simulink model "Flyback75W"  (R2019a)
settings: Solver=VariableStepAuto  StartTime=0.0  StopTime=.05  RelTol=1e-3
libraries: powerlib x21, powerlib_meascontrol x1, simulink x1
settings Model: Creator=victor  LastModifiedBy=victor

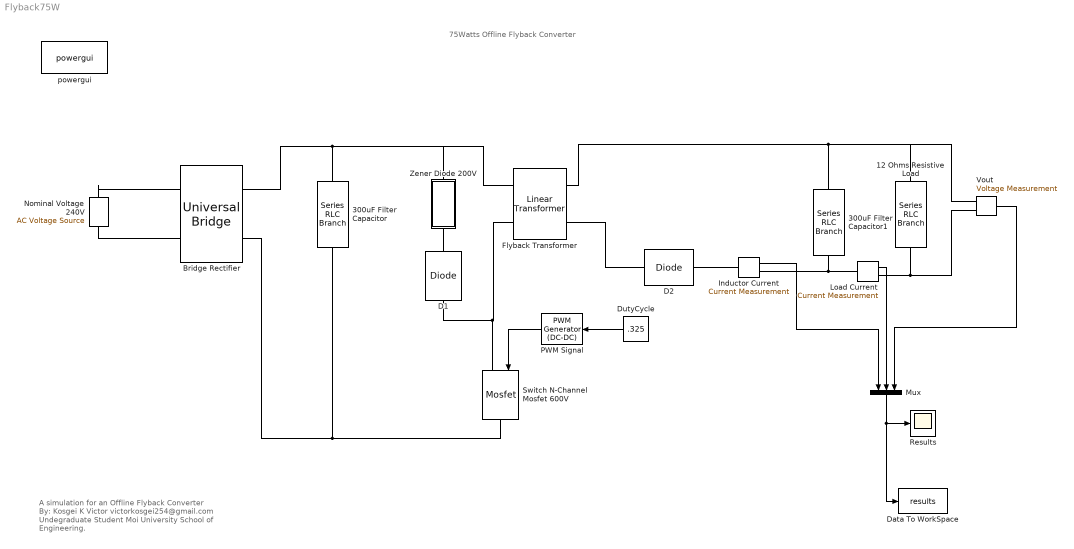
== system Flyback75W ==
  note: 75Watts Offline Flyback Converter
  note: A simulation for an Offline Flyback Converter
      | By: Kosgei K Victor
      | 	victorkosgei254@gmail.com
      | 	Undegraduate Student
      | 	Moi University
      | 	School of Engineering.
  12 Ohms Resistive Load : powerlib/Elements/Series RLC Branch  LConnTagsString=__new0  RConnTagsString=__new0  BranchType=R  Resistance=12  Inductance=1e-3  SetiL0=off  InitialCurrent=0  Capacitance=1e-6  Setx0=off  InitialVoltage=0  Measurements=None
      settings: SourceProductName=Simscape Electrical
  300uF Filter Capacitor : powerlib/Elements/Series RLC Branch  LConnTagsString=__new0  RConnTagsString=__new0  BranchType=C  Resistance=1  Inductance=1e-3  SetiL0=off  InitialCurrent=0  Capacitance=300e-6  Setx0=off  InitialVoltage=0  Measurements=None
      settings: SourceProductName=Simscape Electrical
  300uF Filter Capacitor1 : powerlib/Elements/Series RLC Branch  LConnTagsString=__new0  RConnTagsString=__new0  BranchType=C  Resistance=1  Inductance=1e-3  SetiL0=off  InitialCurrent=0  Capacitance=300e-6  Setx0=off  InitialVoltage=0  Measurements=None
      settings: SourceProductName=Simscape Electrical
  Bridge Rectifier : powerlib/Power Electronics/Universal Bridge  Arms=2  SnubberResistance=1e5  SnubberCapacitance=inf  Device=Diodes  Ron=1e-3  Lon=0  ForwardVoltages="[  0  0  ]"  ForwardVoltage=0  GTOparameters=[ 10e-6 , 20e-6 ]  IGBTparameters=[ 1e-6 , 2e-6 ]  Measurements=None  Measurements_2=None  converterType=Rectifier
      settings: SourceProductName=Simscape Electrical
  D1 : powerlib/Power Electronics/Diode  Ron=0.001  Lon=0  Vf=0.8  IC=0  UseSnubber=0  Rs=500  Cs=250e-9  Measurements=off
      settings: SourceProductName=Simscape Electrical
  D2 : powerlib/Power Electronics/Diode  Ron=0.001  Lon=0  Vf=0.8  IC=0  UseSnubber=0  Rs=500  Cs=250e-9  Measurements=off
      settings: SourceProductName=Simscape Electrical
  Data To WorkSpace : ToWorkspace  VariableName=results  SaveFormat=Timeseries  SampleTime=-1
  DutyCycle : Constant  Value=.325
  Flyback Transformer : powerlib/Elements/Linear Transformer  UNITS=SI  NominalPower=[ 84 250e3 ]  winding1=[540 0 833.9e-6]  winding2=[21.2 0 8.75e-6]  ThreeWindings=off  winding3=[3.15e+05 2.3625e+06 60.161]  RmLm=[3.2156e+12 68.336e-9]  Measurements=None  DataType=on
      settings: SourceProductName=Simscape Electrical
  Inductor Current : powerlib/Measurements/Current Measurement  PhasorSimulation=off  OutputType=Complex  PSBequivalent=0
      settings: SourceProductName=Simscape Electrical
  "Load Current " : powerlib/Measurements/Current Measurement  PhasorSimulation=off  OutputType=Complex  PSBequivalent=0
      settings: SourceProductName=Simscape Electrical
  Mux : Mux  Inputs=3
  Nominal Voltage 240V : powerlib/Electrical Sources/AC Voltage Source  Amplitude=100  Phase=0  Frequency=60  SampleTime=0  Measurements=None  BusType=swing  Pref=10e3  Qref=0  Qmin=-inf  Qmax=+inf
      settings: SourceProductName=Simscape Electrical
  PWM Signal : powerlib_meascontrol/Pulse & Signal Generators/PWM Generator (DC-DC)  Fsw=5000  Ts=0
      settings: SourceProductName=Simscape Electrical
  "Results " : Scope
  Switch N-Channel Mosfet 600V : powerlib/Power Electronics/Mosfet  Ron=0.1  Lon=0  Rd=0.01  Vfd=0  IC=0  Rs=1e5  Cs=inf  Measurements=off
      settings: SourceProductName=Simscape Electrical
  Vout : powerlib/Measurements/Voltage Measurement  PhasorSimulation=off  OutputType=Complex  PSBequivalent=0
      settings: SourceProductName=Simscape Electrical
  Zener Diode 200V : Subsystem  mask(Zener Diode){Vz=10, Rzt=10, Rzk=400, Izm=400e-3, Vf=0.7, Ron=1e-3}
      mask prompts: Vz "Zener Voltage Vz (V)"; Rzt "Dynamic Impedance Zzt (ohms)"; Rzk "Knee Impedance Zzk (ohms)"; Izm "Maximum Continuous Current Izm (A)"; Vf "Forward Voltage Drop Vf (V)"; Ron "On Resistance Ron (ohms)"
      mask help:
      | Implements a zener diode block.
      | Use values from standard datasheets to populate block dialog
  powergui : powerlib/powergui  Priority=1  SimulationMode=Discrete  SampleTime=1e-6  frequency=60  Iterations=50  frequencyindice=60  Pbase=100e6  ErrMax=1e-4  UnitsV=kV  UnitsW=MW  buscounter=0  FunctionMessages=off  echomessages=off  EnableUseOfTLC=off  CurrentSourceSwitches=off  DisableSnubberDevices=off  DisableRonSwitches=off  DisableVfSwitches=off  DisplayEquations=off  AutomaticDiscreteSolvers=off  SolverType=Tustin/Backward Euler (TBE)  Interpol=off  ExternalGateDelay=off  methode=off  Ts=100  x0status=blocks  SPID=on  SwTol=0  HookPort=off  NonlinearTolerance=0  nMaxIteration=15  ContinueOnMaxIteration=off  RestoreLinks=warning  ResistiveCurrentMeasurement=off  Frange=[0:2:500]  Ylog=off  Xlog=on  ShowGrid=off  save=off  variable=ZData  structure=0  ZoomFFT=off  StartTime=0.0  cycles=1  DisplayStyle=1  fundamental=60  FreqAxis=off  MaxFrequency=1000  frequencyindicesteady=1  RmsSteady=1  display=off
      settings: SourceProductName=Simscape Electrical
  wires:
  PWM Signal/1 -> Switch N-Channel Mosfet 600V/1
  DutyCycle/1 -> PWM Signal/1
  Inductor Current/1 -> Mux/1
  "Load Current "/1 -> Mux/2
  Vout/1 -> Mux/3
  Mux/1 -> Data To WorkSpace/1, "Results "/1
  connections:
  Nominal Voltage 240V/RConn1 -- Bridge Rectifier/LConn1
  Nominal Voltage 240V/LConn1 -- Bridge Rectifier/LConn2
  Bridge Rectifier/RConn1 -- Zener Diode 200V/LConn1 -- Flyback Transformer/LConn1 -- 300uF Filter Capacitor/LConn1
  Flyback Transformer/LConn2 -- D1/LConn1 -- Switch N-Channel Mosfet 600V/LConn1
  Switch N-Channel Mosfet 600V/RConn1 -- 300uF Filter Capacitor/RConn1 -- Bridge Rectifier/RConn2
  Flyback Transformer/RConn2 -- D2/LConn1
  Inductor Current/RConn1 -- "Load Current "/LConn1 -- 300uF Filter Capacitor1/LConn1
  Flyback Transformer/RConn1 -- 12 Ohms Resistive Load/RConn1 -- Vout/LConn1 -- 300uF Filter Capacitor1/RConn1
  Inductor Current/LConn1 -- D2/RConn1
  12 Ohms Resistive Load/LConn1 -- Vout/LConn2 -- "Load Current "/RConn1
  Zener Diode 200V/RConn1 -- D1/RConn1

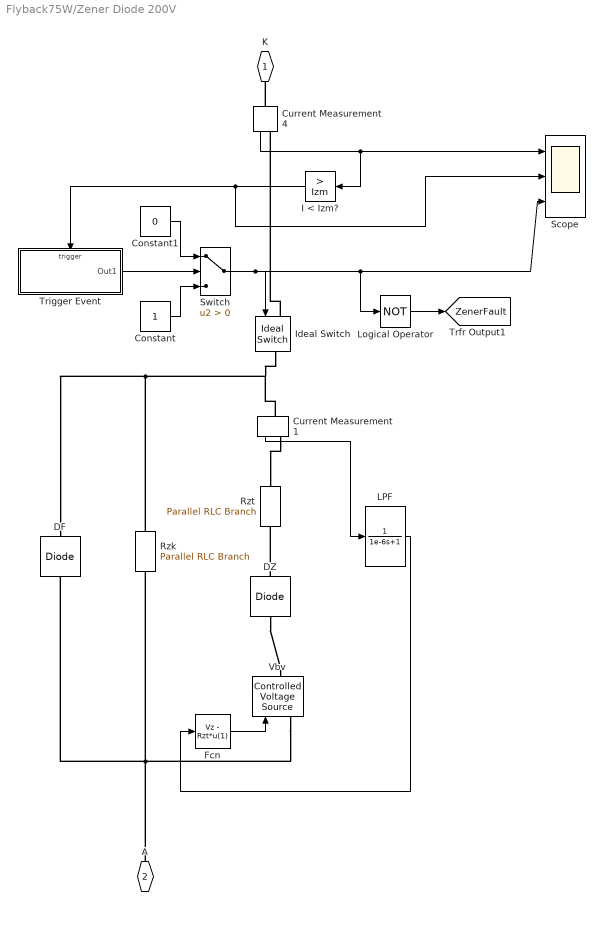
== system Flyback75W/Zener Diode 200V ==
  Constant : Constant
  Constant1 : Constant  Value=0
  Current Measurement1 : powerlib/Measurements/Current Measurement  PhasorSimulation=off  OutputType=Complex  PSBequivalent=0
      settings: SourceProductName=Simscape Electrical
  Current Measurement4 : powerlib/Measurements/Current Measurement  PhasorSimulation=off  OutputType=Complex  PSBequivalent=0
      settings: SourceProductName=Simscape Electrical
  DF : powerlib/Power Electronics/Diode  Ron=Ron  Lon=0  Vf=Vf  IC=0  UseSnubber=off  Rs=1000  Cs=0  Measurements=off
      settings: SourceProductName=Simscape Electrical
  DZ : powerlib/Power Electronics/Diode  Ron=1e-6  Lon=0  Vf=0  IC=0  UseSnubber=off  Rs=100  Cs=inf  Measurements=off
      settings: SourceProductName=Simscape Electrical
  Fcn : Fcn  Expr=Vz - Rzt*u(1)
  I < Izm? : simulink/Logic and Bit Operations/Compare To Constant  relop=>  const=Izm  OutDataTypeStr=boolean
  Ideal Switch : powerlib/Power Electronics/Ideal Switch  Ron=0.001  Lon=0  IC=1  Rs=1e5  Cs=0  Measurements=off
      settings: SourceProductName=Simscape Electrical
  LPF : TransferFcn  Denominator=[1e-6 1]
  Logical Operator : Logic  Operator=NOT  AllPortsSameDT=off  OutDataTypeStr=boolean
  Rzk : powerlib/Elements/Parallel RLC Branch  LConnTagsString=a  RConnTagsString=__new0  BranchType=R  Resistance=Rzk  Inductance=1.0  SetiL0=off  InitialCurrent=0  Capacitance=1e-5  Setx0=off  InitialVoltage=0  Measurements=None
      settings: SourceProductName=Simscape Electrical
  Rzt : powerlib/Elements/Parallel RLC Branch  LConnTagsString=a  RConnTagsString=__new0  BranchType=R  Resistance=Rzt  Inductance=1.0  SetiL0=off  InitialCurrent=0  Capacitance=1e-5  Setx0=off  InitialVoltage=0  Measurements=None
      settings: SourceProductName=Simscape Electrical
  Scope : Scope  NumInputPorts=3
  Switch : Switch  Criteria=u2 > Threshold
  Trigger Event : Subsystem  TreatAsAtomicUnit=on
  Vbv : powerlib/Electrical Sources/Controlled Voltage Source  Initialize=off  Source_Type=DC  Amplitude=0  Phase=0  Frequency=0  Measurements=None
      settings: SourceProductName=Simscape Electrical
  K : PMIOPort  Side=Left
  A : PMIOPort  Port=2  Side=Right
  tag scope: ZenerFault=global
  wires:
  Fcn/1 -> Vbv/1
  Current Measurement4/1 -> Scope/1, I < Izm?/1
  Current Measurement1/1 -> LPF/1
  LPF/1 -> Fcn/1
  I < Izm?/1 -> Scope/2, Trigger Event/Trigger
  Switch/1 -> Ideal Switch/1, Scope/3, Logical Operator/1
  Trigger Event/1(Out1) -> Switch/2
  Constant/1 -> Switch/3
  Constant1/1 -> Switch/1
  Logical Operator/1 -> [ZenerFault]
  connections:
  DZ/RConn1 -- Vbv/RConn1
  Current Measurement4/LConn1 -- K/RConn1
  DZ/LConn1 -- Rzt/LConn1
  Current Measurement1/RConn1 -- Rzt/RConn1
  Rzk/RConn1 -- Current Measurement1/LConn1 -- Ideal Switch/RConn1 -- DF/RConn1
  Ideal Switch/LConn1 -- Current Measurement4/RConn1
  A/RConn1 -- DF/LConn1 -- Rzk/LConn1 -- Vbv/LConn1

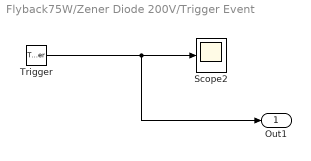
== system Flyback75W/Zener Diode 200V/Trigger Event ==
  Trigger : TriggerPort  VariantControl=Variant  ShowOutputPort=on
  Scope2 : Scope
  Out1 : Outport
  wires:
  Trigger/1 -> Scope2/1, Out1/1
